simulink model "aerodynamics_model"  (R2021a)
settings: Solver=VariableStepAuto  StartTime=0.0  StopTime=10.0  RelTol=1e-3
settings Model: Creator=Nabil  LastModifiedBy=Nabil

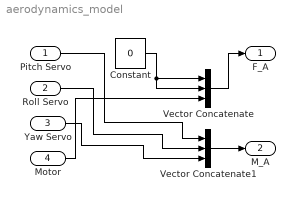
== system aerodynamics_model ==
  Pitch Servo : Inport
  Roll Servo : Inport  Port=2
  Yaw Servo : Inport  Port=3
  Motor : Inport  Port=4
  Constant : Constant  Value=0
  Vector Concatenate : Concatenate  NumInputs=3
  Vector Concatenate1 : Concatenate  NumInputs=3
  F_A : Outport
  M_A : Outport  Port=2
  wires:
  Vector Concatenate/1 -> F_A/1
  Vector Concatenate1/1 -> M_A/1
  Motor/1 -> Vector Concatenate/3
  Pitch Servo/1 -> Vector Concatenate1/1
  Constant/1 -> Vector Concatenate/2, Vector Concatenate/1
  Roll Servo/1 -> Vector Concatenate1/2
  Yaw Servo/1 -> Vector Concatenate1/3
